simulink model "preliminaryModel_noBS13"  (R2015b)
settings: Solver=FixedStepAuto  StartTime=cmd_time(1215)  StopTime=cmd_time(1215)+10  FixedStep=1E-2  MaxStep=0.08  RelTol=1e-3
values from neighbouring files (symbols this model uses):
  act_0 = 0.3    [runfirst13.m]
  b = 1.365    [runfirst13.m]
  cbar = 0.5    [runfirst13.m]
  CD_alpha = 0.173    [runfirst13.m]
  CD_beta = 0    [runfirst13.m]
  CD_ca = 0    [runfirst13.m]
  CD_el = 0    [runfirst13.m]
  CG = [Xcg Ycg Zcg]    [runfirst13.m]
  CL_alpha = 3.137    [runfirst13.m]
  Cl_alpha = 0    [runfirst13.m]
  Cl_beta = 0.046    [runfirst13.m]
  CL_beta = 0    [runfirst13.m]
  CL_ca = 0.000    (= 0)    [runfirst13.m]
  Cl_ca = 0.000    (= 0)    [runfirst13.m]
  CL_el = 0.000    (= 0)    [runfirst13.m]
  Cl_el = 0.111    [runfirst13.m]
  Cm_alpha = -0.083    [runfirst13.m]
  Cm_beta = 0    [runfirst13.m]
  Cm_ca = -0.456    [runfirst13.m]
  Cm_el = 0.000    (= 0)    [runfirst13.m]
  Cn_alpha = 0    [runfirst13.m]
  Cn_beta = 0    [runfirst13.m]
  Cn_ca = 0.000    (= 0)    [runfirst13.m]
  Cn_el = 0.037    [runfirst13.m]
  CP = [xa_ref 0 0]    [runfirst13.m]
  CY_alpha = 0    [runfirst13.m]
  CY_beta = -0.351    [runfirst13.m]
  CY_ca = 0.000    (= 0)    [runfirst13.m]
  CY_el = 0.049    [runfirst13.m]
  deg_2_rad = 1/rad_2_deg    (= 0.0174532925199)    [runfirst13.m]
  eul_0 = [phi_0 theta_0 psi_0]    [runfirst13.m]
  f = 1/196.877360    (= 0.00507930419221)    [runfirst13.m]
  F_0 = [100 0 0]    [runfirst13.m]
  g = 9.82    [runfirst13.m]
  h_ref = 0    [runfirst13.m]
  heading_0 = 0    [runfirst13.m]
  Iyy = 0.01    [runfirst13.m]
  LL0 = [1 0]    [runfirst13.m]
  m_dot = 0.2    [runfirst13.m]
  mass = W_oew    (= 14.95)    [runfirst13.m]
  mass_e = 0    [runfirst13.m]
  mass_f = mass+W_if    (= 17.85)    [runfirst13.m]
  maxdef_act = 2.0    (= 2)    [runfirst13.m]
  maxrate_act = inf    [runfirst13.m]
  mindef_act = -2.0    (= -2)    [runfirst13.m]
  P_g = 100000    [runfirst13.m]
  pos3_0 = [Xe_0 Ze_0]    [runfirst13.m]
  pos_0 = [Xe_0 Ye_0 Ze_0]    [runfirst13.m]
  q_0 = 0.5    [runfirst13.m]
  R = 287    [runfirst13.m]
  rad_2_deg = 180/pi    (= 57.2957795131)    [runfirst13.m]
  rho_ref = 1.225    [runfirst13.m]
  rot_0 = [p_0 q_0 r_0]    [runfirst13.m]
  S_ref = 0.747    [runfirst13.m]
  T_g = 293    [runfirst13.m]
  theta_0 = 0.02    [runfirst13.m]
  U_0 = 10    [runfirst13.m]
  Vb_0 = [U_0 v_0 w_0]    [runfirst13.m]
  Vw_0 = [uw_0 vw_0 ww_0]    [runfirst13.m]
  w_0 = 0    [runfirst13.m]
  wn_act = 1.7    [runfirst13.m]
  z_act = 0.57    [runfirst13.m]
undefined symbols (not defined in the file or in its folder): Newton, Raphson, U0, w0
libraries: simulink x6
(part 2 of 2)

== system preliminaryModel_noBS13/Aerodynamics/Control stab/Subsystem/Canard ==
  note: in airspeed
  note: use mder_ca/elp/els/ru and take incoming angles to sink? and just run the values cause they go same timestepNUMBER, not timeseries objects
      | when running own piloting take angles and just gain BUT CHECK CORRECT EQUATION SO ITS ACTUALLY THE DERIVATIVES
  In1 : Inport
  CD : Gain  Gain=CD_ca  SaturateOnIntegerOverflow=on  OutDataTypeStr=Inherit: Same as input  ParamDataTypeStr=Inherit: Same as input
  CL : Gain  Gain=CL_ca  SaturateOnIntegerOverflow=on  OutDataTypeStr=Inherit: Same as input  ParamDataTypeStr=Inherit: Same as input
  CY : Gain  Gain=CY_ca  SaturateOnIntegerOverflow=on  OutDataTypeStr=Inherit: Same as input  ParamDataTypeStr=Inherit: Same as input
  Cl : Gain  Gain=Cl_ca  SaturateOnIntegerOverflow=on  OutDataTypeStr=Inherit: Same as input  ParamDataTypeStr=Inherit: Same as input
  Cm : Gain  Gain=Cm_ca  SaturateOnIntegerOverflow=on  OutDataTypeStr=Inherit: Same as input  ParamDataTypeStr=Inherit: Same as input
  Cn : Gain  Gain=Cn_ca  SaturateOnIntegerOverflow=on  OutDataTypeStr=Inherit: Same as input  ParamDataTypeStr=Inherit: Same as input
  Mux1 : Mux  Inputs=6
  DerivCanard : Outport
  wires:
  CY/1 -> Mux1/2  "CY"
  Cl/1 -> Mux1/4  "Cl"
  CD/1 -> Mux1/1  "CD"
  Cm/1 -> Mux1/5  "Cm"
  Cn/1 -> Mux1/6  "Cn"
  In1/1 -> Cn/1, Cm/1, Cl/1, CL/1, CY/1, CD/1
  CL/1 -> Mux1/3  "CL"
  Mux1/1 -> DerivCanard/1

== system preliminaryModel_noBS13/Aerodynamics/Control stab/Subsystem/Elevon 1  ==
  In1 : Inport
  CD : Gain  Gain=CD_el  SaturateOnIntegerOverflow=on  OutDataTypeStr=Inherit: Same as input  ParamDataTypeStr=Inherit: Same as input
  CL : Gain  Gain=CL_el  SaturateOnIntegerOverflow=on  OutDataTypeStr=Inherit: Same as input  ParamDataTypeStr=Inherit: Same as input
  CY : Gain  Gain=CY_el  SaturateOnIntegerOverflow=on  OutDataTypeStr=Inherit: Same as input  ParamDataTypeStr=Inherit: Same as input
  Cl : Gain  Gain=Cl_el  SaturateOnIntegerOverflow=on  OutDataTypeStr=Inherit: Same as input  ParamDataTypeStr=Inherit: Same as input
  Cm : Gain  Gain=Cm_el  SaturateOnIntegerOverflow=on  OutDataTypeStr=Inherit: Same as input  ParamDataTypeStr=Inherit: Same as input
  Cn : Gain  Gain=Cn_el  SaturateOnIntegerOverflow=on  OutDataTypeStr=Inherit: Same as input  ParamDataTypeStr=Inherit: Same as input
  Mux1 : Mux  Inputs=6
  DerivElevonPort : Outport
  wires:
  CY/1 -> Mux1/2  "CY"
  Cl/1 -> Mux1/4  "Cl"
  CD/1 -> Mux1/1  "CD"
  Cm/1 -> Mux1/5  "Cm"
  Cn/1 -> Mux1/6  "Cn"
  In1/1 -> Cn/1, Cm/1, Cl/1, CL/1, CY/1, CD/1
  CL/1 -> Mux1/3  "CL"
  Mux1/1 -> DerivElevonPort/1

== system preliminaryModel_noBS13/Aerodynamics/Control stab/Subsystem/Elevon 2  ==
  In1 : Inport
  CD : Gain  Gain=CD_el  SaturateOnIntegerOverflow=on  OutDataTypeStr=Inherit: Same as input  ParamDataTypeStr=Inherit: Same as input
  CL : Gain  Gain=CL_el  SaturateOnIntegerOverflow=on  OutDataTypeStr=Inherit: Same as input  ParamDataTypeStr=Inherit: Same as input
  CY : Gain  Gain=CY_el  SaturateOnIntegerOverflow=on  OutDataTypeStr=Inherit: Same as input  ParamDataTypeStr=Inherit: Same as input
  Cl : Gain  Gain=Cl_el  SaturateOnIntegerOverflow=on  OutDataTypeStr=Inherit: Same as input  ParamDataTypeStr=Inherit: Same as input
  Cm : Gain  Gain=Cm_el  SaturateOnIntegerOverflow=on  OutDataTypeStr=Inherit: Same as input  ParamDataTypeStr=Inherit: Same as input
  Cn : Gain  Gain=Cn_el  SaturateOnIntegerOverflow=on  OutDataTypeStr=Inherit: Same as input  ParamDataTypeStr=Inherit: Same as input
  Mux1 : Mux  Inputs=6
  DerivElevonStar : Outport
  wires:
  CY/1 -> Mux1/2  "CY"
  Cl/1 -> Mux1/4  "Cl"
  CD/1 -> Mux1/1  "CD"
  Cm/1 -> Mux1/5  "Cm"
  Cn/1 -> Mux1/6  "Cn"
  In1/1 -> Cn/1, Cm/1, Cl/1, CL/1, CY/1, CD/1
  CL/1 -> Mux1/3  "CL"
  Mux1/1 -> DerivElevonStar/1

== system preliminaryModel_noBS13/Aerodynamics/Control stab/Subsystem/Rudder  ==
  In1 : Inport
  CD : Gain  Gain=0  SaturateOnIntegerOverflow=on  OutDataTypeStr=Inherit: Same as input  ParamDataTypeStr=Inherit: Same as input
  CL : Gain  Gain=Cm_ca  SaturateOnIntegerOverflow=on  OutDataTypeStr=Inherit: Same as input  ParamDataTypeStr=Inherit: Same as input
  CY : Gain  Gain=CL_ca  SaturateOnIntegerOverflow=on  OutDataTypeStr=Inherit: Same as input  ParamDataTypeStr=Inherit: Same as input
  Cl : Gain  Gain=Cm_ca  SaturateOnIntegerOverflow=on  OutDataTypeStr=Inherit: Same as input  ParamDataTypeStr=Inherit: Same as input
  Cm : Gain  Gain=Cm_ca  SaturateOnIntegerOverflow=on  OutDataTypeStr=Inherit: Same as input  ParamDataTypeStr=Inherit: Same as input
  Cn : Gain  Gain=Cm_ca  SaturateOnIntegerOverflow=on  OutDataTypeStr=Inherit: Same as input  ParamDataTypeStr=Inherit: Same as input
  Mux1 : Mux  Inputs=6
  DerivRudder : Outport
  wires:
  CY/1 -> Mux1/2  "CY"
  Cl/1 -> Mux1/4  "Cl"
  CD/1 -> Mux1/1  "CD"
  Cm/1 -> Mux1/5  "Cm"
  Cn/1 -> Mux1/6  "Cn"
  In1/1 -> Cn/1, Cm/1, Cl/1, CL/1, CY/1, CD/1
  CL/1 -> Mux1/3  "CL"
  Mux1/1 -> DerivRudder/1

== system preliminaryModel_noBS13/Aerodynamics/Subsystem5/3x3 Cross Product/Subsystem1 ==
  A : Inport
  B : Inport  Port=2
  Demux : Demux  Outputs=3
  Demux1 : Demux  Outputs=3
  Mux : Mux  Inputs=3
  i x j : Product  SaturateOnIntegerOverflow=on  InputSameDT=on  OutDataTypeStr=Inherit: Same as first input
  j x k : Product  SaturateOnIntegerOverflow=on  InputSameDT=on  OutDataTypeStr=Inherit: Same as first input
  k x i : Product  SaturateOnIntegerOverflow=on  InputSameDT=on  OutDataTypeStr=Inherit: Same as first input
  Out1 : Outport
  wires:
  Demux1/3 -> j x k/2
  Demux/2 -> j x k/1
  Demux/3 -> k x i/1
  Demux1/1 -> k x i/2
  Demux1/2 -> i x j/2
  Demux/1 -> i x j/1
  i x j/1 -> Mux/3
  k x i/1 -> Mux/2
  j x k/1 -> Mux/1
  B/1 -> Demux1/1
  A/1 -> Demux/1
  Mux/1 -> Out1/1

== system preliminaryModel_noBS13/Aerodynamics/Subsystem5/3x3 Cross Product/Subsystem3 ==
  A : Inport
  B : Inport  Port=2
  Demux : Demux  Outputs=3
  Demux1 : Demux  Outputs=3
  Mux : Mux  Inputs=3
  i x k : Product  SaturateOnIntegerOverflow=on  InputSameDT=on  OutDataTypeStr=Inherit: Same as first input
  j x i : Product  SaturateOnIntegerOverflow=on  InputSameDT=on  OutDataTypeStr=Inherit: Same as first input
  k x j : Product  SaturateOnIntegerOverflow=on  InputSameDT=on  OutDataTypeStr=Inherit: Same as first input
  Out1 : Outport
  wires:
  j x i/1 -> Mux/3
  i x k/1 -> Mux/2
  k x j/1 -> Mux/1
  Mux/1 -> Out1/1
  Demux1/1 -> j x i/2
  Demux/2 -> j x i/1
  Demux1/3 -> i x k/2
  Demux/1 -> i x k/1
  Demux1/2 -> k x j/2
  Demux/3 -> k x j/1
  B/1 -> Demux1/1
  A/1 -> Demux/1

== system preliminaryModel_noBS13/Aerodynamics/Subsystem5/Subsystem/Subsystem ==
  alpha beta : Inport  PortDimensions=2
  A11 : Subsystem
  A12 : Subsystem
  A13 : Subsystem
  A21 : Subsystem
  A22 : Subsystem
  A23 : Subsystem
  A31 : Subsystem
  A32 : Subsystem
  A33 : Subsystem
  Mux1 : Mux  Inputs=2
  Subsystem : Subsystem
  sincos : Trigonometry  Operator=sincos
  DCM : Outport  PortDimensions=[3,3]  InitialOutput=0
  wires:
  A21/1(A21) -> Subsystem/4(M21)
  Mux1/1 -> A23/1(sin_cos), A32/1(sin_cos), A33/1(sin_cos), A31/1(sin_cos), A22/1(sin_cos), A12/1(sin_cos), A11/1(sin_cos), A13/1(sin_cos), A21/1(sin_cos)
  A23/1(A23) -> Subsystem/6(M23)
  A31/1(A31) -> Subsystem/7(M31)
  A32/1(A32) -> Subsystem/8(M32)
  A22/1(A22) -> Subsystem/5(M22)
  alpha beta/1 -> sincos/1
  sincos/2 -> Mux1/2
  A13/1(A13) -> Subsystem/3(M13)
  A11/1(A11) -> Subsystem/1(M11)
  A33/1(A33) -> Subsystem/9(M33)
  sincos/1 -> Mux1/1
  Subsystem/1(Matrix) -> DCM/1
  A12/1(A12) -> Subsystem/2(M12)

== system preliminaryModel_noBS13/Aerodynamics/Subsystem5/Subsystem/Subsystem1 ==
  Vb : Inport
  "Airspeed " : Sqrt  AlgorithmType=Newton-Raphson  SaturateOnIntegerOverflow=on
  "Indicence  " : Trigonometry  Operator=atan2
  Product1 : Product  Inputs=*/  SaturateOnIntegerOverflow=on  OutDataTypeStr=Inherit: Same as first input
  Sideslip : Trigonometry  Operator=asin
  Subsystem1 : Subsystem
  Subsystem3 : Subsystem
  Subsystem4 : Subsystem
  Alpha : Outport
  Beta : Outport  Port=2
  V : Outport  Port=3
  wires:
  Subsystem4/2(U) -> "Indicence  "/2
  Subsystem4/1(w) -> "Indicence  "/1
  "Airspeed "/1 -> V/1, Product1/2
  Sideslip/1 -> Beta/1
  Subsystem3/1(v) -> Product1/1
  Subsystem1/1(dot) -> "Airspeed "/1
  Vb/1 -> Subsystem1/1(Vb), Subsystem3/1(Vb), Subsystem4/1(Vb)
  "Indicence  "/1 -> Alpha/1
  Product1/1 -> Sideslip/1

== system preliminaryModel_noBS13/Aerodynamics/Subsystem5/Subsystem2/Subsystem ==
  alpha beta : Inport  PortDimensions=2
  A11 : Subsystem
  A12 : Subsystem
  A13 : Subsystem
  A21 : Subsystem
  A22 : Subsystem
  A23 : Subsystem
  A31 : Subsystem
  A32 : Subsystem
  A33 : Subsystem
  Mux1 : Mux  Inputs=2
  Subsystem : Subsystem
  sincos : Trigonometry  Operator=sincos
  DCM : Outport  PortDimensions=[3,3]  InitialOutput=0
  wires:
  A21/1(A21) -> Subsystem/4(M21)
  Mux1/1 -> A22/1(sin_cos), A23/1(sin_cos), A31/1(sin_cos), A32/1(sin_cos), A33/1(sin_cos), A21/1(sin_cos), A13/1(sin_cos), A12/1(sin_cos), A11/1(sin_cos)
  A31/1(A31) -> Subsystem/7(M31)
  A23/1(A23) -> Subsystem/6(M23)
  A32/1(A32) -> Subsystem/8(M32)
  A22/1(A22) -> Subsystem/5(M22)
  alpha beta/1 -> sincos/1
  sincos/2 -> Mux1/2
  A13/1(A13) -> Subsystem/3(M13)
  A11/1(A11) -> Subsystem/1(M11)
  A33/1(A33) -> Subsystem/9(M33)
  sincos/1 -> Mux1/1
  Subsystem/1(Matrix) -> DCM/1
  A12/1(A12) -> Subsystem/2(M12)

== system preliminaryModel_noBS13/Aerodynamics/Subsystem5/Subsystem2/Subsystem1 ==
  Vb : Inport
  "Airspeed " : Sqrt  AlgorithmType=Newton-Raphson  SaturateOnIntegerOverflow=on
  "Indicence  " : Trigonometry  Operator=atan2
  Product1 : Product  Inputs=*/  SaturateOnIntegerOverflow=on  OutDataTypeStr=Inherit: Same as first input
  Sideslip : Trigonometry  Operator=asin
  Subsystem1 : Subsystem
  Subsystem3 : Subsystem
  Subsystem4 : Subsystem
  Alpha : Outport
  Beta : Outport  Port=2
  V : Outport  Port=3
  wires:
  Subsystem4/2(U) -> "Indicence  "/2
  Subsystem4/1(w) -> "Indicence  "/1
  "Airspeed "/1 -> V/1, Product1/2
  Sideslip/1 -> Beta/1
  Subsystem3/1(v) -> Product1/1
  Subsystem1/1(dot) -> "Airspeed "/1
  Vb/1 -> Subsystem1/1(Vb), Subsystem3/1(Vb), Subsystem4/1(Vb)
  "Indicence  "/1 -> Alpha/1
  Product1/1 -> Sideslip/1

== system preliminaryModel_noBS13/Aerodynamics/Subsystem5/Subsystem3/Subsystem ==
  alpha beta : Inport  PortDimensions=2
  A11 : Subsystem
  A12 : Subsystem
  A13 : Subsystem
  A21 : Subsystem
  A22 : Subsystem
  A23 : Subsystem
  A31 : Subsystem
  A32 : Subsystem
  A33 : Subsystem
  Mux1 : Mux  Inputs=2
  Subsystem : Subsystem
  sincos : Trigonometry  Operator=sincos
  DCM : Outport  PortDimensions=[3,3]  InitialOutput=0
  wires:
  A21/1(A21) -> Subsystem/4(M21)
  Mux1/1 -> A22/1(sin_cos), A23/1(sin_cos), A31/1(sin_cos), A32/1(sin_cos), A33/1(sin_cos), A21/1(sin_cos), A13/1(sin_cos), A12/1(sin_cos), A11/1(sin_cos)
  A31/1(A31) -> Subsystem/7(M31)
  A23/1(A23) -> Subsystem/6(M23)
  A32/1(A32) -> Subsystem/8(M32)
  A22/1(A22) -> Subsystem/5(M22)
  alpha beta/1 -> sincos/1
  sincos/2 -> Mux1/2
  A13/1(A13) -> Subsystem/3(M13)
  A11/1(A11) -> Subsystem/1(M11)
  A33/1(A33) -> Subsystem/9(M33)
  sincos/1 -> Mux1/1
  Subsystem/1(Matrix) -> DCM/1
  A12/1(A12) -> Subsystem/2(M12)

== system preliminaryModel_noBS13/Aerodynamics/Subsystem5/Subsystem3/Subsystem1 ==
  Vb : Inport
  "Airspeed " : Sqrt  AlgorithmType=Newton-Raphson  SaturateOnIntegerOverflow=on
  "Indicence  " : Trigonometry  Operator=atan2
  Product1 : Product  Inputs=*/  SaturateOnIntegerOverflow=on  OutDataTypeStr=Inherit: Same as first input
  Sideslip : Trigonometry  Operator=asin
  Subsystem1 : Subsystem
  Subsystem3 : Subsystem
  Subsystem4 : Subsystem
  Alpha : Outport
  Beta : Outport  Port=2
  V : Outport  Port=3
  wires:
  Subsystem4/2(U) -> "Indicence  "/2
  Subsystem4/1(w) -> "Indicence  "/1
  "Airspeed "/1 -> V/1, Product1/2
  Sideslip/1 -> Beta/1
  Subsystem3/1(v) -> Product1/1
  Subsystem1/1(dot) -> "Airspeed "/1
  Vb/1 -> Subsystem1/1(Vb), Subsystem3/1(Vb), Subsystem4/1(Vb)
  "Indicence  "/1 -> Alpha/1
  Product1/1 -> Sideslip/1

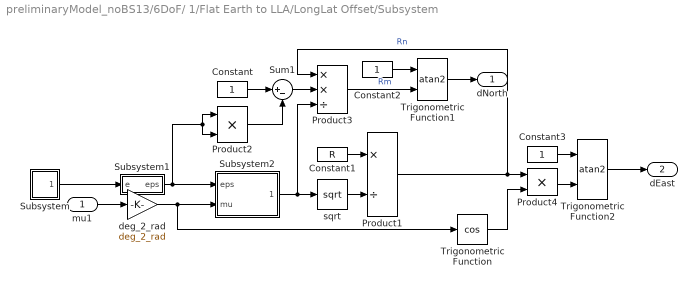
== system preliminaryModel_noBS13/6DoF/ 1/Flat Earth to LLA/LongLat Offset/Subsystem ==
  mu1 : Inport
  Constant : Constant
  Constant1 : Constant  Value=R
  Constant2 : Constant
  Constant3 : Constant
  Product1 : Product  Inputs=*/  RndMeth=Zero
  Product2 : Product  RndMeth=Zero
  Product3 : Product  Inputs=**/  RndMeth=Zero
  Product4 : Product  RndMeth=Zero
  Subsystem : Subsystem
  Subsystem1 : Subsystem
  Subsystem2 : Subsystem
  Sum1 : Sum  Inputs=|+-
  Trigonometric Function : Trigonometry  Operator=cos
  Trigonometric Function1 : Trigonometry  Operator=atan2
  Trigonometric Function2 : Trigonometry  Operator=atan2
  deg_2_rad : Gain  Gain=deg_2_rad
  sqrt : Sqrt  AlgorithmType=Newton-Raphson  SaturateOnIntegerOverflow=on
  dNorth : Outport
  dEast : Outport  Port=2
  wires:
  Trigonometric Function1/1 -> dNorth/1
  Subsystem/1(e1) -> Subsystem1/1(e)
  Subsystem2/1(denom1) -> sqrt/1, Product3/3
  Subsystem1/1(eps) -> Subsystem2/1(eps), Product2/2, Product2/1
  Constant1/1 -> Product1/1
  sqrt/1 -> Product1/2
  Constant/1 -> Sum1/1
  Product2/1 -> Sum1/2
  Product1/1 -> Product4/1, Product3/1  "Rn"
  Sum1/1 -> Product3/2
  Product3/1 -> Trigonometric Function1/2  "Rm"
  Trigonometric Function/1 -> Product4/2
  mu1/1 -> deg_2_rad/1
  Product4/1 -> Trigonometric Function2/2
  Constant3/1 -> Trigonometric Function2/1
  Constant2/1 -> Trigonometric Function1/1
  deg_2_rad/1 -> Subsystem2/2(mu), Trigonometric Function/1
  Trigonometric Function2/1 -> dEast/1

== system preliminaryModel_noBS13/6DoF/ 1/Flat Earth to LLA/Subsystem/Latitude Wrap 90 ==
  Lat : Inport
  Abs1 : Abs
  Bias : Bias  Bias=-90
  Bias1 : Bias  Bias=+90
  Compare To Constant : simulink/Logic and Bit Operations/Compare To Constant  relop=>  const=90  OutDataTypeStr=boolean
  Divide1 : Product  Inputs=**
  Gain : Gain  Gain=-1
  Sign1 : Signum
  Switch : Switch  Criteria=u2 ~= 0
  Wrap Angle 180 : Subsystem
  Lat wrapped : Outport
  Wrap flag : Outport  Port=2
  wires:
  Compare To Constant/1 -> Switch/2, Wrap flag/1
  Wrap Angle 180/1(Angle 180) -> Sign1/1, Switch/3, Abs1/1
  Lat/1 -> Wrap Angle 180/1(Angle)
  Abs1/1 -> Compare To Constant/1, Bias/1
  Bias/1 -> Gain/1
  Gain/1 -> Bias1/1
  Bias1/1 -> Divide1/2
  Sign1/1 -> Divide1/1
  Divide1/1 -> Switch/1
  Switch/1 -> Lat wrapped/1

== system preliminaryModel_noBS13/6DoF/ 1/Flat Earth to LLA/Subsystem/Wrap Longitude ==
  Angle : Inport
  Abs : Abs
  Bias : Bias  Bias=180
  Bias1 : Bias  Bias=-180
  Compare To Constant : simulink/Logic and Bit Operations/Compare To Constant  relop=>  const=180  OutDataTypeStr=boolean
  Constant2 : Constant  Value=360
  Math Function1 : Math  Operator=mod  SaturateOnIntegerOverflow=on
  Switch : Switch  Criteria=u2 ~= 0  Threshold=180
  Angle 180 : Outport
  wires:
  Compare To Constant/1 -> Switch/2
  Angle/1 -> Bias/1, Switch/3, Abs/1
  Abs/1 -> Compare To Constant/1
  Bias/1 -> Math Function1/1
  Constant2/1 -> Math Function1/2
  Math Function1/1 -> Bias1/1
  Bias1/1 -> Switch/1
  Switch/1 -> Angle 180/1

== system preliminaryModel_noBS13/6DoF/ 1/Flat Earth to LLA/Subsystem1/Latitude Wrap 90 ==
  Lat : Inport
  Abs1 : Abs
  Bias : Bias  Bias=-90
  Bias1 : Bias  Bias=+90
  Compare To Constant : simulink/Logic and Bit Operations/Compare To Constant  relop=>  const=90  OutDataTypeStr=boolean
  Divide1 : Product  Inputs=**
  Gain : Gain  Gain=-1
  Sign1 : Signum
  Switch : Switch  Criteria=u2 ~= 0
  Wrap Angle 180 : Subsystem
  Lat wrapped : Outport
  Wrap flag : Outport  Port=2
  wires:
  Compare To Constant/1 -> Switch/2, Wrap flag/1
  Wrap Angle 180/1(Angle 180) -> Sign1/1, Switch/3, Abs1/1
  Lat/1 -> Wrap Angle 180/1(Angle)
  Abs1/1 -> Compare To Constant/1, Bias/1
  Bias/1 -> Gain/1
  Gain/1 -> Bias1/1
  Bias1/1 -> Divide1/2
  Sign1/1 -> Divide1/1
  Divide1/1 -> Switch/1
  Switch/1 -> Lat wrapped/1

== system preliminaryModel_noBS13/6DoF/ 1/Flat Earth to LLA/Subsystem1/Wrap Longitude ==
  Angle : Inport
  Abs : Abs
  Bias : Bias  Bias=180
  Bias1 : Bias  Bias=-180
  Compare To Constant : simulink/Logic and Bit Operations/Compare To Constant  relop=>  const=180  OutDataTypeStr=boolean
  Constant2 : Constant  Value=360
  Math Function1 : Math  Operator=mod  SaturateOnIntegerOverflow=on
  Switch : Switch  Criteria=u2 ~= 0  Threshold=180
  Angle 180 : Outport
  wires:
  Compare To Constant/1 -> Switch/2
  Angle/1 -> Bias/1, Switch/3, Abs/1
  Abs/1 -> Compare To Constant/1
  Bias/1 -> Math Function1/1
  Constant2/1 -> Math Function1/2
  Math Function1/1 -> Bias1/1
  Bias1/1 -> Switch/1
  Switch/1 -> Angle 180/1

== system preliminaryModel_noBS13/6DoF/6DOF/Calculate omega_dot/wx(Iw)/Subsystem ==
  A : Inport
  B : Inport  Port=2
  Demux : Demux  Outputs=3
  Demux1 : Demux  Outputs=3
  Mux : Mux  Inputs=3
  i x j : Product  SaturateOnIntegerOverflow=on  InputSameDT=on  OutDataTypeStr=Inherit: Same as first input
  j x k : Product  SaturateOnIntegerOverflow=on  InputSameDT=on  OutDataTypeStr=Inherit: Same as first input
  k x i : Product  SaturateOnIntegerOverflow=on  InputSameDT=on  OutDataTypeStr=Inherit: Same as first input
  Out1 : Outport
  wires:
  Demux1/3 -> j x k/2
  Demux/2 -> j x k/1
  Demux/3 -> k x i/1
  Demux1/1 -> k x i/2
  Demux1/2 -> i x j/2
  Demux/1 -> i x j/1
  i x j/1 -> Mux/3
  k x i/1 -> Mux/2
  j x k/1 -> Mux/1
  B/1 -> Demux1/1
  A/1 -> Demux/1
  Mux/1 -> Out1/1

== system preliminaryModel_noBS13/6DoF/6DOF/Calculate omega_dot/wx(Iw)/Subsystem1 ==
  A : Inport
  B : Inport  Port=2
  Demux : Demux  Outputs=3
  Demux1 : Demux  Outputs=3
  Mux : Mux  Inputs=3
  i x k : Product  SaturateOnIntegerOverflow=on  InputSameDT=on  OutDataTypeStr=Inherit: Same as first input
  j x i : Product  SaturateOnIntegerOverflow=on  InputSameDT=on  OutDataTypeStr=Inherit: Same as first input
  k x j : Product  SaturateOnIntegerOverflow=on  InputSameDT=on  OutDataTypeStr=Inherit: Same as first input
  Out1 : Outport
  wires:
  j x i/1 -> Mux/3
  i x k/1 -> Mux/2
  k x j/1 -> Mux/1
  Mux/1 -> Out1/1
  Demux1/1 -> j x i/2
  Demux/2 -> j x i/1
  Demux1/3 -> i x k/2
  Demux/1 -> i x k/1
  Demux1/2 -> k x j/2
  Demux/3 -> k x j/1
  B/1 -> Demux1/1
  A/1 -> Demux/1

== system preliminaryModel_noBS13/6DoF/6DOF/Subsystem/Rotation Angles to Direction Cosine Matrix/Subsystem ==
  M11 : Inport  PortDimensions=1
  M12 : Inport  Port=2  PortDimensions=1
  M13 : Inport  Port=3  PortDimensions=1
  M21 : Inport  Port=4  PortDimensions=1
  M22 : Inport  Port=5  PortDimensions=1
  M23 : Inport  Port=6  PortDimensions=1
  M31 : Inport  Port=7  PortDimensions=1
  M32 : Inport  Port=8  PortDimensions=1
  M33 : Inport  Port=9  PortDimensions=1
  Reshape (9) to [3x3] column-major : Reshape  OutputDimensionality=Customize  OutputDimensions=[3,3]
  Vector Concatenate : Concatenate  NumInputs=9
  Matrix : Outport  PortDimensions=[3 3]
  wires:
  M33/1 -> Vector Concatenate/9
  M21/1 -> Vector Concatenate/2
  Vector Concatenate/1 -> Reshape (9) to [3x3] column-major/1
  M11/1 -> Vector Concatenate/1
  M31/1 -> Vector Concatenate/3
  M12/1 -> Vector Concatenate/4
  M22/1 -> Vector Concatenate/5
  Reshape (9) to [3x3] column-major/1 -> Matrix/1
  M32/1 -> Vector Concatenate/6
  M13/1 -> Vector Concatenate/7
  M23/1 -> Vector Concatenate/8

== system preliminaryModel_noBS13/Aerodynamics/Subsystem5/Subsystem/Subsystem/A11 ==
  sin_cos : Inport
  Demux : Demux  Outputs=2
  Selector : Selector  InputPortWidth=4  IndexOptions=Index vector (dialog)  Indices=[3 4 ]  OutputSizes=1
  u(3)*u(4) : Product  RndMeth=Zero
  A11 : Outport
  wires:
  Demux/2 -> u(3)*u(4)/2
  Demux/1 -> u(3)*u(4)/1
  Selector/1 -> Demux/1
  u(3)*u(4)/1 -> A11/1
  sin_cos/1 -> Selector/1

== system preliminaryModel_noBS13/Aerodynamics/Subsystem5/Subsystem/Subsystem/A12 ==
  sin_cos : Inport
  Selector : Selector  InputPortWidth=4  IndexOptions=Index vector (dialog)  Indices=2  OutputSizes=1
  A12 : Outport
  wires:
  Selector/1 -> A12/1
  sin_cos/1 -> Selector/1

== system preliminaryModel_noBS13/Aerodynamics/Subsystem5/Subsystem/Subsystem/A13 ==
  sin_cos : Inport
  Demux : Demux  Outputs=2
  Selector : Selector  InputPortWidth=4  IndexOptions=Index vector (dialog)  Indices=[1 4 ]  OutputSizes=1
  u(1)*u(4) : Product  RndMeth=Zero
  A13 : Outport
  wires:
  Selector/1 -> Demux/1
  Demux/2 -> u(1)*u(4)/2
  Demux/1 -> u(1)*u(4)/1
  sin_cos/1 -> Selector/1
  u(1)*u(4)/1 -> A13/1

== system preliminaryModel_noBS13/Aerodynamics/Subsystem5/Subsystem/Subsystem/A21 ==
  sin_cos : Inport
  Demux : Demux  Outputs=2
  Selector : Selector  InputPortWidth=4  IndexOptions=Index vector (dialog)  Indices=[2 3 ]  OutputSizes=1
  Unary Minus : UnaryMinus
  u(2)*u(3) : Product  RndMeth=Zero
  A21 : Outport
  wires:
  Selector/1 -> Demux/1
  Demux/2 -> u(2)*u(3)/2
  Demux/1 -> u(2)*u(3)/1
  Unary Minus/1 -> A21/1
  sin_cos/1 -> Selector/1
  u(2)*u(3)/1 -> Unary Minus/1

== system preliminaryModel_noBS13/Aerodynamics/Subsystem5/Subsystem/Subsystem/A22 ==
  sin_cos : Inport
  Selector : Selector  InputPortWidth=4  IndexOptions=Index vector (dialog)  Indices=4  OutputSizes=1
  A22 : Outport
  wires:
  Selector/1 -> A22/1
  sin_cos/1 -> Selector/1

== system preliminaryModel_noBS13/Aerodynamics/Subsystem5/Subsystem/Subsystem/A23 ==
  sin_cos : Inport
  Demux : Demux  Outputs=2
  Selector : Selector  InputPortWidth=4  IndexOptions=Index vector (dialog)  Indices=[1 2]  OutputSizes=1
  Unary Minus : UnaryMinus
  u(1)*u(2) : Product  RndMeth=Zero
  A23 : Outport
  wires:
  Selector/1 -> Demux/1
  u(1)*u(2)/1 -> Unary Minus/1
  sin_cos/1 -> Selector/1
  Demux/1 -> u(1)*u(2)/1
  Demux/2 -> u(1)*u(2)/2
  Unary Minus/1 -> A23/1

== system preliminaryModel_noBS13/Aerodynamics/Subsystem5/Subsystem/Subsystem/A31 ==
  sin_cos : Inport
  Selector : Selector  InputPortWidth=4  IndexOptions=Index vector (dialog)  Indices=1  OutputSizes=1
  Unary Minus : UnaryMinus
  A31 : Outport
  wires:
  Selector/1 -> Unary Minus/1
  Unary Minus/1 -> A31/1
  sin_cos/1 -> Selector/1

== system preliminaryModel_noBS13/Aerodynamics/Subsystem5/Subsystem/Subsystem/A32 ==
  sin_cos : Inport
  Constant : Constant  Value=0
  Terminator3 : Terminator
  A32 : Outport
  wires:
  sin_cos/1 -> Terminator3/1
  Constant/1 -> A32/1

== system preliminaryModel_noBS13/Aerodynamics/Subsystem5/Subsystem/Subsystem/A33 ==
  sin_cos : Inport
  Selector : Selector  InputPortWidth=4  IndexOptions=Index vector (dialog)  Indices=3  OutputSizes=1
  A33 : Outport
  wires:
  Selector/1 -> A33/1
  sin_cos/1 -> Selector/1

== system preliminaryModel_noBS13/Aerodynamics/Subsystem5/Subsystem/Subsystem/Subsystem ==
  M11 : Inport  PortDimensions=1
  M12 : Inport  Port=2  PortDimensions=1
  M13 : Inport  Port=3  PortDimensions=1
  M21 : Inport  Port=4  PortDimensions=1
  M22 : Inport  Port=5  PortDimensions=1
  M23 : Inport  Port=6  PortDimensions=1
  M31 : Inport  Port=7  PortDimensions=1
  M32 : Inport  Port=8  PortDimensions=1
  M33 : Inport  Port=9  PortDimensions=1
  Reshape (9) to [3x3] column-major : Reshape  OutputDimensionality=Customize  OutputDimensions=[3,3]
  Vector Concatenate : Concatenate  NumInputs=9
  Matrix : Outport  PortDimensions=[3 3]
  wires:
  M23/1 -> Vector Concatenate/8
  M12/1 -> Vector Concatenate/4
  M33/1 -> Vector Concatenate/9
  Reshape (9) to [3x3] column-major/1 -> Matrix/1
  M22/1 -> Vector Concatenate/5
  M13/1 -> Vector Concatenate/7
  M11/1 -> Vector Concatenate/1
  M21/1 -> Vector Concatenate/2
  Vector Concatenate/1 -> Reshape (9) to [3x3] column-major/1
  M31/1 -> Vector Concatenate/3
  M32/1 -> Vector Concatenate/6

== system preliminaryModel_noBS13/Aerodynamics/Subsystem5/Subsystem/Subsystem1/Subsystem1 ==
  Vb : Inport
  Demux1 : Demux  Outputs=3
  Product : Product  RndMeth=Zero
  Product1 : Product  RndMeth=Zero
  Product2 : Product  RndMeth=Zero
  Sum : Sum  Inputs=+++
  dot : Outport
  wires:
  Product1/1 -> Sum/2
  Product/1 -> Sum/1
  Demux1/1 -> Product/2, Product/1
  Vb/1 -> Demux1/1
  Sum/1 -> dot/1
  Demux1/2 -> Product1/1, Product1/2
  Demux1/3 -> Product2/2, Product2/1
  Product2/1 -> Sum/3

== system preliminaryModel_noBS13/Aerodynamics/Subsystem5/Subsystem/Subsystem1/Subsystem3 ==
  Vb : Inport
  Demux1 : Demux  Outputs=3
  Terminator : Terminator
  Terminator1 : Terminator
  v : Outport
  wires:
  Demux1/1 -> Terminator/1
  Demux1/3 -> Terminator1/1
  Vb/1 -> Demux1/1
  Demux1/2 -> v/1

== system preliminaryModel_noBS13/Aerodynamics/Subsystem5/Subsystem/Subsystem1/Subsystem4 ==
  Vb : Inport
  Demux1 : Demux  Outputs=3
  Terminator : Terminator
  w : Outport
  U : Outport  Port=2
  wires:
  Demux1/2 -> Terminator/1
  Demux1/3 -> w/1
  Vb/1 -> Demux1/1
  Demux1/1 -> U/1

== system preliminaryModel_noBS13/Aerodynamics/Subsystem5/Subsystem2/Subsystem/A11 ==
  sin_cos : Inport
  Demux : Demux  Outputs=2
  Selector : Selector  InputPortWidth=4  IndexOptions=Index vector (dialog)  Indices=[3 4 ]  OutputSizes=1
  u(3)*u(4) : Product  RndMeth=Zero
  A11 : Outport
  wires:
  Demux/2 -> u(3)*u(4)/2
  Demux/1 -> u(3)*u(4)/1
  Selector/1 -> Demux/1
  u(3)*u(4)/1 -> A11/1
  sin_cos/1 -> Selector/1

== system preliminaryModel_noBS13/Aerodynamics/Subsystem5/Subsystem2/Subsystem/A12 ==
  sin_cos : Inport
  Selector : Selector  InputPortWidth=4  IndexOptions=Index vector (dialog)  Indices=2  OutputSizes=1
  A12 : Outport
  wires:
  Selector/1 -> A12/1
  sin_cos/1 -> Selector/1

== system preliminaryModel_noBS13/Aerodynamics/Subsystem5/Subsystem2/Subsystem/A13 ==
  sin_cos : Inport
  Demux : Demux  Outputs=2
  Selector : Selector  InputPortWidth=4  IndexOptions=Index vector (dialog)  Indices=[1 4 ]  OutputSizes=1
  u(1)*u(4) : Product  RndMeth=Zero
  A13 : Outport
  wires:
  Selector/1 -> Demux/1
  Demux/2 -> u(1)*u(4)/2
  Demux/1 -> u(1)*u(4)/1
  sin_cos/1 -> Selector/1
  u(1)*u(4)/1 -> A13/1

== system preliminaryModel_noBS13/Aerodynamics/Subsystem5/Subsystem2/Subsystem/A21 ==
  sin_cos : Inport
  Demux : Demux  Outputs=2
  Selector : Selector  InputPortWidth=4  IndexOptions=Index vector (dialog)  Indices=[2 3 ]  OutputSizes=1
  Unary Minus : UnaryMinus
  u(2)*u(3) : Product  RndMeth=Zero
  A21 : Outport
  wires:
  Selector/1 -> Demux/1
  Demux/2 -> u(2)*u(3)/2
  Demux/1 -> u(2)*u(3)/1
  Unary Minus/1 -> A21/1
  sin_cos/1 -> Selector/1
  u(2)*u(3)/1 -> Unary Minus/1

== system preliminaryModel_noBS13/Aerodynamics/Subsystem5/Subsystem2/Subsystem/A22 ==
  sin_cos : Inport
  Selector : Selector  InputPortWidth=4  IndexOptions=Index vector (dialog)  Indices=4  OutputSizes=1
  A22 : Outport
  wires:
  Selector/1 -> A22/1
  sin_cos/1 -> Selector/1

== system preliminaryModel_noBS13/Aerodynamics/Subsystem5/Subsystem2/Subsystem/A23 ==
  sin_cos : Inport
  Demux : Demux  Outputs=2
  Selector : Selector  InputPortWidth=4  IndexOptions=Index vector (dialog)  Indices=[1 2]  OutputSizes=1
  Unary Minus : UnaryMinus
  u(1)*u(2) : Product  RndMeth=Zero
  A23 : Outport
  wires:
  Selector/1 -> Demux/1
  u(1)*u(2)/1 -> Unary Minus/1
  sin_cos/1 -> Selector/1
  Demux/1 -> u(1)*u(2)/1
  Demux/2 -> u(1)*u(2)/2
  Unary Minus/1 -> A23/1

== system preliminaryModel_noBS13/Aerodynamics/Subsystem5/Subsystem2/Subsystem/A31 ==
  sin_cos : Inport
  Selector : Selector  InputPortWidth=4  IndexOptions=Index vector (dialog)  Indices=1  OutputSizes=1
  Unary Minus : UnaryMinus
  A31 : Outport
  wires:
  Selector/1 -> Unary Minus/1
  Unary Minus/1 -> A31/1
  sin_cos/1 -> Selector/1

== system preliminaryModel_noBS13/Aerodynamics/Subsystem5/Subsystem2/Subsystem/A32 ==
  sin_cos : Inport
  Constant : Constant  Value=0
  Terminator3 : Terminator
  A32 : Outport
  wires:
  sin_cos/1 -> Terminator3/1
  Constant/1 -> A32/1

== system preliminaryModel_noBS13/Aerodynamics/Subsystem5/Subsystem2/Subsystem/A33 ==
  sin_cos : Inport
  Selector : Selector  InputPortWidth=4  IndexOptions=Index vector (dialog)  Indices=3  OutputSizes=1
  A33 : Outport
  wires:
  Selector/1 -> A33/1
  sin_cos/1 -> Selector/1

== system preliminaryModel_noBS13/Aerodynamics/Subsystem5/Subsystem2/Subsystem/Subsystem ==
  M11 : Inport  PortDimensions=1
  M12 : Inport  Port=2  PortDimensions=1
  M13 : Inport  Port=3  PortDimensions=1
  M21 : Inport  Port=4  PortDimensions=1
  M22 : Inport  Port=5  PortDimensions=1
  M23 : Inport  Port=6  PortDimensions=1
  M31 : Inport  Port=7  PortDimensions=1
  M32 : Inport  Port=8  PortDimensions=1
  M33 : Inport  Port=9  PortDimensions=1
  Reshape (9) to [3x3] column-major : Reshape  OutputDimensionality=Customize  OutputDimensions=[3,3]
  Vector Concatenate : Concatenate  NumInputs=9
  Matrix : Outport  PortDimensions=[3 3]
  wires:
  M23/1 -> Vector Concatenate/8
  M12/1 -> Vector Concatenate/4
  M33/1 -> Vector Concatenate/9
  Reshape (9) to [3x3] column-major/1 -> Matrix/1
  M22/1 -> Vector Concatenate/5
  M13/1 -> Vector Concatenate/7
  M11/1 -> Vector Concatenate/1
  M21/1 -> Vector Concatenate/2
  Vector Concatenate/1 -> Reshape (9) to [3x3] column-major/1
  M31/1 -> Vector Concatenate/3
  M32/1 -> Vector Concatenate/6

== system preliminaryModel_noBS13/Aerodynamics/Subsystem5/Subsystem2/Subsystem1/Subsystem1 ==
  Vb : Inport
  Demux1 : Demux  Outputs=3
  Product : Product  RndMeth=Zero
  Product1 : Product  RndMeth=Zero
  Product2 : Product  RndMeth=Zero
  Sum : Sum  Inputs=+++
  dot : Outport
  wires:
  Product1/1 -> Sum/2
  Product/1 -> Sum/1
  Demux1/1 -> Product/2, Product/1
  Vb/1 -> Demux1/1
  Sum/1 -> dot/1
  Demux1/2 -> Product1/1, Product1/2
  Demux1/3 -> Product2/2, Product2/1
  Product2/1 -> Sum/3

== system preliminaryModel_noBS13/Aerodynamics/Subsystem5/Subsystem2/Subsystem1/Subsystem3 ==
  Vb : Inport
  Demux1 : Demux  Outputs=3
  Terminator : Terminator
  Terminator1 : Terminator
  v : Outport
  wires:
  Demux1/1 -> Terminator/1
  Demux1/3 -> Terminator1/1
  Vb/1 -> Demux1/1
  Demux1/2 -> v/1

== system preliminaryModel_noBS13/Aerodynamics/Subsystem5/Subsystem2/Subsystem1/Subsystem4 ==
  Vb : Inport
  Demux1 : Demux  Outputs=3
  Terminator : Terminator
  w : Outport
  U : Outport  Port=2
  wires:
  Demux1/2 -> Terminator/1
  Demux1/3 -> w/1
  Vb/1 -> Demux1/1
  Demux1/1 -> U/1

== system preliminaryModel_noBS13/Aerodynamics/Subsystem5/Subsystem3/Subsystem/A11 ==
  sin_cos : Inport
  Demux : Demux  Outputs=2
  Selector : Selector  InputPortWidth=4  IndexOptions=Index vector (dialog)  Indices=[3 4 ]  OutputSizes=1
  u(3)*u(4) : Product  RndMeth=Zero
  A11 : Outport
  wires:
  Demux/2 -> u(3)*u(4)/2
  Demux/1 -> u(3)*u(4)/1
  Selector/1 -> Demux/1
  u(3)*u(4)/1 -> A11/1
  sin_cos/1 -> Selector/1

== system preliminaryModel_noBS13/Aerodynamics/Subsystem5/Subsystem3/Subsystem/A12 ==
  sin_cos : Inport
  Selector : Selector  InputPortWidth=4  IndexOptions=Index vector (dialog)  Indices=2  OutputSizes=1
  A12 : Outport
  wires:
  Selector/1 -> A12/1
  sin_cos/1 -> Selector/1

== system preliminaryModel_noBS13/Aerodynamics/Subsystem5/Subsystem3/Subsystem/A13 ==
  sin_cos : Inport
  Demux : Demux  Outputs=2
  Selector : Selector  InputPortWidth=4  IndexOptions=Index vector (dialog)  Indices=[1 4 ]  OutputSizes=1
  u(1)*u(4) : Product  RndMeth=Zero
  A13 : Outport
  wires:
  Selector/1 -> Demux/1
  Demux/2 -> u(1)*u(4)/2
  Demux/1 -> u(1)*u(4)/1
  sin_cos/1 -> Selector/1
  u(1)*u(4)/1 -> A13/1

== system preliminaryModel_noBS13/Aerodynamics/Subsystem5/Subsystem3/Subsystem/A21 ==
  sin_cos : Inport
  Demux : Demux  Outputs=2
  Selector : Selector  InputPortWidth=4  IndexOptions=Index vector (dialog)  Indices=[2 3 ]  OutputSizes=1
  Unary Minus : UnaryMinus
  u(2)*u(3) : Product  RndMeth=Zero
  A21 : Outport
  wires:
  Selector/1 -> Demux/1
  Demux/2 -> u(2)*u(3)/2
  Demux/1 -> u(2)*u(3)/1
  Unary Minus/1 -> A21/1
  sin_cos/1 -> Selector/1
  u(2)*u(3)/1 -> Unary Minus/1

== system preliminaryModel_noBS13/Aerodynamics/Subsystem5/Subsystem3/Subsystem/A22 ==
  sin_cos : Inport
  Selector : Selector  InputPortWidth=4  IndexOptions=Index vector (dialog)  Indices=4  OutputSizes=1
  A22 : Outport
  wires:
  Selector/1 -> A22/1
  sin_cos/1 -> Selector/1

== system preliminaryModel_noBS13/Aerodynamics/Subsystem5/Subsystem3/Subsystem/A23 ==
  sin_cos : Inport
  Demux : Demux  Outputs=2
  Selector : Selector  InputPortWidth=4  IndexOptions=Index vector (dialog)  Indices=[1 2]  OutputSizes=1
  Unary Minus : UnaryMinus
  u(1)*u(2) : Product  RndMeth=Zero
  A23 : Outport
  wires:
  Selector/1 -> Demux/1
  u(1)*u(2)/1 -> Unary Minus/1
  sin_cos/1 -> Selector/1
  Demux/1 -> u(1)*u(2)/1
  Demux/2 -> u(1)*u(2)/2
  Unary Minus/1 -> A23/1

== system preliminaryModel_noBS13/Aerodynamics/Subsystem5/Subsystem3/Subsystem/A31 ==
  sin_cos : Inport
  Selector : Selector  InputPortWidth=4  IndexOptions=Index vector (dialog)  Indices=1  OutputSizes=1
  Unary Minus : UnaryMinus
  A31 : Outport
  wires:
  Selector/1 -> Unary Minus/1
  Unary Minus/1 -> A31/1
  sin_cos/1 -> Selector/1

== system preliminaryModel_noBS13/Aerodynamics/Subsystem5/Subsystem3/Subsystem/A32 ==
  sin_cos : Inport
  Constant : Constant  Value=0
  Terminator3 : Terminator
  A32 : Outport
  wires:
  sin_cos/1 -> Terminator3/1
  Constant/1 -> A32/1

== system preliminaryModel_noBS13/Aerodynamics/Subsystem5/Subsystem3/Subsystem/A33 ==
  sin_cos : Inport
  Selector : Selector  InputPortWidth=4  IndexOptions=Index vector (dialog)  Indices=3  OutputSizes=1
  A33 : Outport
  wires:
  Selector/1 -> A33/1
  sin_cos/1 -> Selector/1

== system preliminaryModel_noBS13/Aerodynamics/Subsystem5/Subsystem3/Subsystem/Subsystem ==
  M11 : Inport  PortDimensions=1
  M12 : Inport  Port=2  PortDimensions=1
  M13 : Inport  Port=3  PortDimensions=1
  M21 : Inport  Port=4  PortDimensions=1
  M22 : Inport  Port=5  PortDimensions=1
  M23 : Inport  Port=6  PortDimensions=1
  M31 : Inport  Port=7  PortDimensions=1
  M32 : Inport  Port=8  PortDimensions=1
  M33 : Inport  Port=9  PortDimensions=1
  Reshape (9) to [3x3] column-major : Reshape  OutputDimensionality=Customize  OutputDimensions=[3,3]
  Vector Concatenate : Concatenate  NumInputs=9
  Matrix : Outport  PortDimensions=[3 3]
  wires:
  M23/1 -> Vector Concatenate/8
  M12/1 -> Vector Concatenate/4
  M33/1 -> Vector Concatenate/9
  Reshape (9) to [3x3] column-major/1 -> Matrix/1
  M22/1 -> Vector Concatenate/5
  M13/1 -> Vector Concatenate/7
  M11/1 -> Vector Concatenate/1
  M21/1 -> Vector Concatenate/2
  Vector Concatenate/1 -> Reshape (9) to [3x3] column-major/1
  M31/1 -> Vector Concatenate/3
  M32/1 -> Vector Concatenate/6

== system preliminaryModel_noBS13/Aerodynamics/Subsystem5/Subsystem3/Subsystem1/Subsystem1 ==
  Vb : Inport
  Demux1 : Demux  Outputs=3
  Product : Product  RndMeth=Zero
  Product1 : Product  RndMeth=Zero
  Product2 : Product  RndMeth=Zero
  Sum : Sum  Inputs=+++
  dot : Outport
  wires:
  Product1/1 -> Sum/2
  Product/1 -> Sum/1
  Demux1/1 -> Product/2, Product/1
  Vb/1 -> Demux1/1
  Sum/1 -> dot/1
  Demux1/2 -> Product1/1, Product1/2
  Demux1/3 -> Product2/2, Product2/1
  Product2/1 -> Sum/3

== system preliminaryModel_noBS13/Aerodynamics/Subsystem5/Subsystem3/Subsystem1/Subsystem3 ==
  Vb : Inport
  Demux1 : Demux  Outputs=3
  Terminator : Terminator
  Terminator1 : Terminator
  v : Outport
  wires:
  Demux1/1 -> Terminator/1
  Demux1/3 -> Terminator1/1
  Vb/1 -> Demux1/1
  Demux1/2 -> v/1

== system preliminaryModel_noBS13/Aerodynamics/Subsystem5/Subsystem3/Subsystem1/Subsystem4 ==
  Vb : Inport
  Demux1 : Demux  Outputs=3
  Terminator : Terminator
  w : Outport
  U : Outport  Port=2
  wires:
  Demux1/2 -> Terminator/1
  Demux1/3 -> w/1
  Vb/1 -> Demux1/1
  Demux1/1 -> U/1

== system preliminaryModel_noBS13/6DoF/ 1/Flat Earth to LLA/LongLat Offset/Subsystem/Subsystem ==
  Constant4 : Constant  Value=f
  Sum : Sum  Inputs=-+
  f : Constant
  e1 : Outport
  wires:
  Sum/1 -> e1/1
  f/1 -> Sum/2
  Constant4/1 -> Sum/1

== system preliminaryModel_noBS13/6DoF/ 1/Flat Earth to LLA/LongLat Offset/Subsystem/Subsystem1 ==
  e : Inport
  Constant4 : Constant
  Product5 : Product  RndMeth=Zero
  Sum2 : Sum  Inputs=|+-
  sqrt1 : Sqrt  AlgorithmType=Newton-Raphson  SaturateOnIntegerOverflow=on
  eps : Outport
  wires:
  Sum2/1 -> sqrt1/1
  Product5/1 -> Sum2/2
  sqrt1/1 -> eps/1
  Constant4/1 -> Sum2/1
  e/1 -> Product5/1, Product5/2

== system preliminaryModel_noBS13/6DoF/ 1/Flat Earth to LLA/LongLat Offset/Subsystem/Subsystem2 ==
  eps : Inport
  mu : Inport  Port=2
  Constant4 : Constant
  Product5 : Product  Inputs=4  RndMeth=Zero
  Sum2 : Sum  Inputs=|+-
  Trigonometric Function3 : Trigonometry
  denom1 : Outport
  wires:
  Trigonometric Function3/1 -> Product5/4, Product5/3
  Constant4/1 -> Sum2/1
  Sum2/1 -> denom1/1
  eps/1 -> Product5/1, Product5/2
  Product5/1 -> Sum2/2
  mu/1 -> Trigonometric Function3/1

== system preliminaryModel_noBS13/6DoF/ 1/Flat Earth to LLA/Subsystem/Latitude Wrap 90/Wrap Angle 180 ==
  Angle : Inport
  Abs : Abs
  Bias : Bias  Bias=180
  Bias1 : Bias  Bias=-180
  Compare To Constant : simulink/Logic and Bit Operations/Compare To Constant  relop=>  const=180  OutDataTypeStr=boolean
  Constant2 : Constant  Value=360
  Math Function1 : Math  Operator=mod  SaturateOnIntegerOverflow=on
  Switch : Switch  Criteria=u2 ~= 0  Threshold=180
  Angle 180 : Outport
  wires:
  Compare To Constant/1 -> Switch/2
  Angle/1 -> Bias/1, Switch/3, Abs/1
  Abs/1 -> Compare To Constant/1
  Bias/1 -> Math Function1/1
  Constant2/1 -> Math Function1/2
  Math Function1/1 -> Bias1/1
  Bias1/1 -> Switch/1
  Switch/1 -> Angle 180/1

== system preliminaryModel_noBS13/6DoF/ 1/Flat Earth to LLA/Subsystem1/Latitude Wrap 90/Wrap Angle 180 ==
  Angle : Inport
  Abs : Abs
  Bias : Bias  Bias=180
  Bias1 : Bias  Bias=-180
  Compare To Constant : simulink/Logic and Bit Operations/Compare To Constant  relop=>  const=180  OutDataTypeStr=boolean
  Constant2 : Constant  Value=360
  Math Function1 : Math  Operator=mod  SaturateOnIntegerOverflow=on
  Switch : Switch  Criteria=u2 ~= 0  Threshold=180
  Angle 180 : Outport
  wires:
  Compare To Constant/1 -> Switch/2
  Angle/1 -> Bias/1, Switch/3, Abs/1
  Abs/1 -> Compare To Constant/1
  Bias/1 -> Math Function1/1
  Constant2/1 -> Math Function1/2
  Math Function1/1 -> Bias1/1
  Bias1/1 -> Switch/1
  Switch/1 -> Angle 180/1
